simulink model "pendule_inverse"  (R2016a)
settings: Solver=FixedStepAuto  StartTime=0.0  StopTime=100  FixedStep=0.01  RelTol=1e-3
undefined symbols (not defined in the file): sigbuilder_block
libraries: simulink x1
settings Model: Creator=nsurbayr  LastModifiedBy=nsurbayr

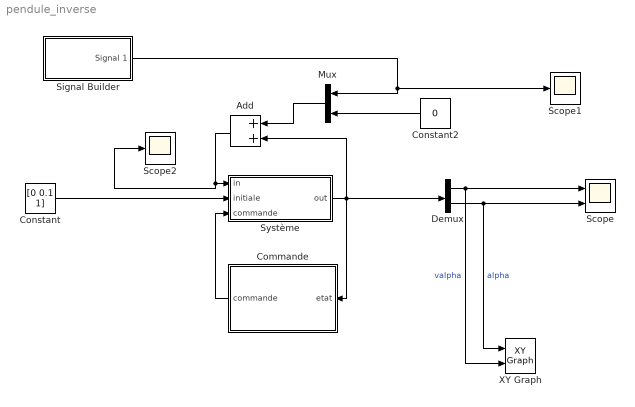
== system pendule_inverse ==
  Add : Sum
  Commande : Subsystem
  Constant : Constant  Value=[0 0.1 1]
  Constant2 : Constant  Value=0
  Demux : Demux  Outputs=2
  Mux : Mux  Inputs=2
  Scope : Scope  NumInputPorts=2
  Scope1 : Scope
  Scope2 : Scope
  Signal Builder : Subsystem  Tag=STV Subsys  LoadFcn=sigbuilder_block('load',[665.432 184.168 563.116 385.011 ]);  StartFcn=sigbuilder_block('start');  StopFcn=sigbuilder_block('stop');  ClipboardFcn=sigbuilder_block('clipboard');  mask(Sigbuilder block){}
      mask help: Simulink:masks:SigbuilderBlock_MD
      mask init:
      | if ~strcmp(get_param(bdroot(gcbh),'SimulationStatus'),'stopped') tuvar = sigbuilder_block('maskInit'); end
      settings: CopyFcn=sigbuilder_block('copy');  DeleteFcn=sigbuilder_block('delete');  ModelCloseFcn=sigbuilder_block('modelClose');  PreSaveFcn=sigbuilder_block('preSave');  PauseFcn=sigbuilder_block('pause');  ContinueFcn=sigbuilder_block('continue');  NameChangeFcn=sigbuilder_block('namechange');  OpenFcn=sigbuilder_block('open',[437.305 199.326 550.989 400.168 ]);  CloseFcn=sigbuilder_block('close');
      mask Display: plot(0, 0, 100, 100,[2, 2, 32, 32, 2], [68, 8, 8, 68, 68],[32, 2], [38, 38], [32, 19, 2],[53, 60, 44], [32, 17, 17, 2],[16, 16, 31, 31]);txt = getActiveGroup(gcbh);text(2, 100, txt,'verticalAlignment', 'top');
  Système : Subsystem
  XY Graph : simulink/Sinks/XY Graph  xmin=-50  xmax=20  ymin=-5  ymax=5  st=-1
  wires:
  Système/1(out) -> Commande/1(etat), Add/2, Demux/1
  Constant/1 -> Système/2(initiale)
  Demux/2 -> XY Graph/1, Scope/2  "alpha"
  Demux/1 -> XY Graph/2, Scope/1  "valpha"
  Add/1 -> Scope2/1, Système/1(in)
  Signal Builder/1(Signal 1) -> Mux/1, Scope1/1
  Mux/1 -> Add/1
  Constant2/1 -> Mux/2
  Commande/1(commande) -> Système/3(commande)

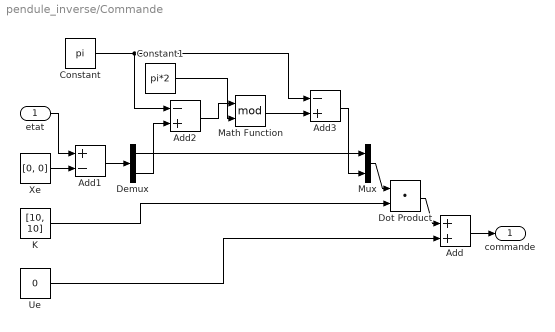
== system pendule_inverse/Commande ==
  etat : Inport
  Add : Sum
  Add1 : Sum  Inputs=+-
  Add2 : Sum  Inputs=-+
  Add3 : Sum  Inputs=-+
  Constant : Constant  Value=pi
  Constant1 : Constant  Value=pi*2
  Demux : Demux  Outputs=2
  Dot Product : DotProduct  InputSameDT=on  OutDataTypeStr=Inherit: Inherit via internal rule
  K : Constant  Value=[10, 10]
  Math Function : Math  Operator=mod  SaturateOnIntegerOverflow=on
  Mux : Mux  Inputs=2
  Ue : Constant  Value=0
  Xe : Constant  Value=[0, 0]
  commande : Outport
  wires:
  Add/1 -> commande/1
  Ue/1 -> Add/2
  Dot Product/1 -> Add/1
  K/1 -> Dot Product/2
  Xe/1 -> Add1/2
  etat/1 -> Add1/1
  Add1/1 -> Demux/1
  Mux/1 -> Dot Product/1
  Demux/1 -> Mux/1
  Add2/1 -> Math Function/1
  Add3/1 -> Mux/2
  Math Function/1 -> Add3/2
  Demux/2 -> Add2/2
  Constant/1 -> Add3/1, Add2/1
  Constant1/1 -> Math Function/2

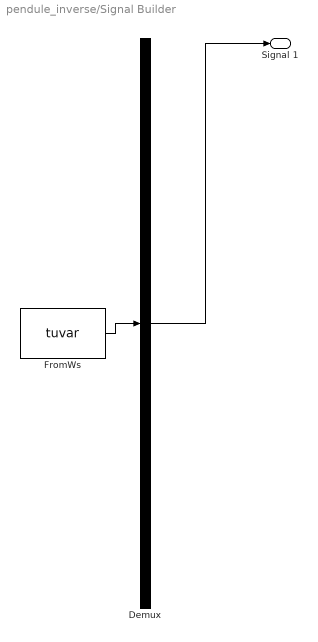
== system pendule_inverse/Signal Builder ==
  Demux : Demux  Tag=STV Demux  Outputs=1
  FromWs : FromWorkspace  Tag=STV FromWs  VariableName=tuvar  SampleTime=0
      SigBuilderData=|
      | common.afterFinalStr = 'Extrapolate'
      | common.sampleTime = 0
      | dataSet.timeRange = [0 100]
      | dataSet.name = 'Group 1'
      | sbobj.Groups.Name = 'Group 1'
      | sbobj.Groups.Signals.Name = 'Signal 1'
      | sbobj.Groups.Signals.XData = [0 58.2 58.2 59.2 59.2 100]
      | sbobj.Groups.Signals.YData = [0 0 3.79 3.79 0 0]
      | sbobj.Groups.TimeRange = [0 100]
  Signal 1 : Outport  Tag=STV Outport
  wires:
  Demux/1 -> Signal 1/1
  FromWs/1 -> Demux/1

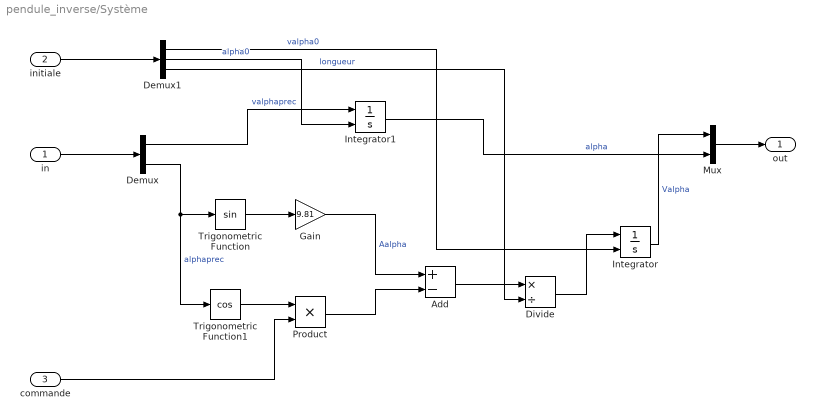
== system pendule_inverse/Système ==
  in : Inport
  initiale : Inport  Port=2
  commande : Inport  Port=3
  Add : Sum  Inputs=+-
  Demux : Demux  Outputs=2
  Demux1 : Demux  Outputs=3
  Divide : Product  Inputs=*/
  Gain : Gain  Gain=9.81
  Integrator : Integrator  InitialConditionSource=external
  Integrator1 : Integrator  InitialConditionSource=external  InitialCondition=pi
  Mux : Mux  Inputs=2
  Product : Product
  Trigonometric Function : Trigonometry
  Trigonometric Function1 : Trigonometry  Operator=cos
  out : Outport
  wires:
  Trigonometric Function/1 -> Gain/1
  in/1 -> Demux/1
  Demux/2 -> Trigonometric Function1/1, Trigonometric Function/1  "alphaprec"
  Mux/1 -> out/1
  Integrator1/1 -> Mux/2  "alpha"
  Integrator/1 -> Mux/1  "Valpha"
  Demux/1 -> Integrator1/1  "valphaprec"
  initiale/1 -> Demux1/1
  Demux1/2 -> Integrator1/2  "alpha0"
  Demux1/1 -> Integrator/2  "valpha0"
  Gain/1 -> Add/1  "Aalpha"
  Divide/1 -> Integrator/1
  Add/1 -> Divide/1
  Demux1/3 -> Divide/2  "longueur"
  Product/1 -> Add/2
  Trigonometric Function1/1 -> Product/1
  commande/1 -> Product/2
